simulink model "polysync_simulink"  (R2017a)
settings: Solver=FixedStepDiscrete  StartTime=0.0  StopTime=10.0  FixedStep=0.01  RelTol=1e-3
libraries: simulink x1, PolySyncLibrary x1
settings Model: Creator=laptopuser  LastModifiedBy=laptopuser
settings DataIOCC: SaveOutput=off  SignalLogging=off  DSMLogging=off  SaveTime=off
settings OptimizationCC: DefaultParameterBehavior=Inlined  UseDivisionForNetSlopeComputation=on  UseFloatMulNetSlope=on  InlineInvariantSignals=on  PassReuseOutputArgsThreshold=0  EfficientFloat2IntCast=on
settings DebuggingCC: ParameterTunabilityLossMsg=error
settings HardwareCC: ProdBitPerLong=64  ProdHWDeviceType=Intel->x86-64 (Linux 64)
settings SFSimCC: SimCustomHeaderCode="#include \"MwPsTypes.hpp\""  MATLABDynamicMemAlloc=off
settings RTWCC: GenerateReport=on  BuildConfiguration=Debug  LaunchReport=on  TargetLang=C++
settings CodeAppCC: ForceParamTrailComments=on  OperatorAnnotations=on  MATLABSourceComments=on
settings GRTTargetCC: TargetLangStandard=C++03 (ISO)

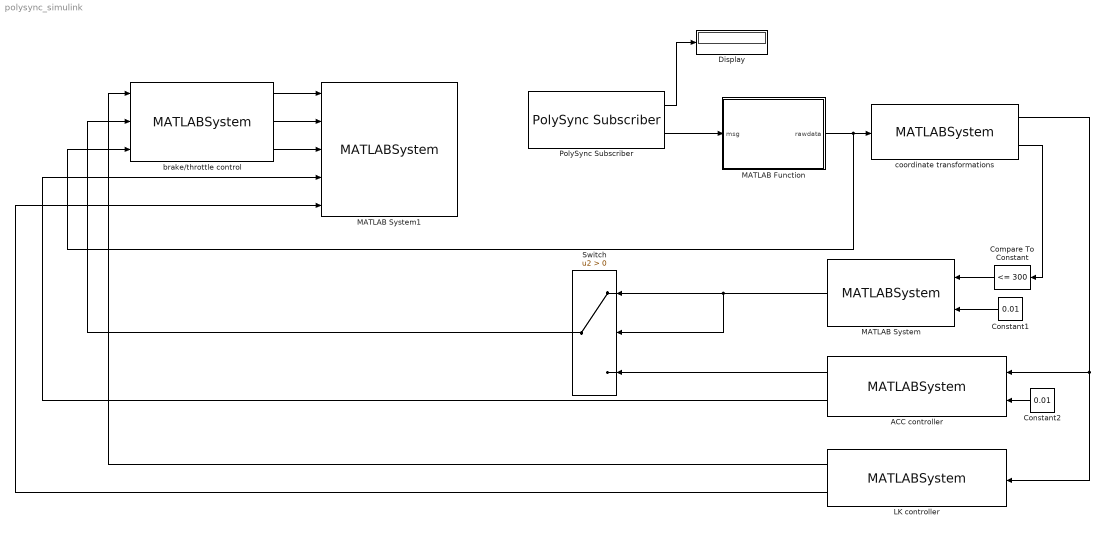
== system polysync_simulink ==
  ACC controller : MATLABSystem  System=acc_pcis_controller  M=1800  f0bar=74.63  f1bar=40.59  vl=26/3.6  v_des=28/3.6  H_x=diag([1 0.001])  f_x=[-28/3.6;0]  H_u=0.0001  f_u=0  K_i=50  sol_opts=struct( 'DataType', 'double', 'MaxIter', 200, 'FeasibilityTol', 1e-6, 'IntegrityChecks', true )  SimulateUsing=Code generation
      mask Type: acc_pcis_controller
      mask Display:
      | disp('acc_pcis_controller');
      | port_label('input',1,'lk_acc_state');
      | port_label('input',2,'dt');
      | port_label('output',1,'F_w');
      | port_label('output',2,'control_info');
  Compare To Constant : simulink/Logic and Bit Operations/Compare To Constant  relop=<=  const=300  OutDataTypeStr=boolean
  Constant1 : Constant  Value=0.01
  Constant2 : Constant  Value=0.01
  Display : Display
  LK controller : MATLABSystem  System=lk_pcis_controller  M=1800  lf=1.2  lr=1.650  Caf=140000  Car=120000  Iz=3270.0  H_x=diag([1 0 0.5 0])  f_x=[0;0;0;0]  H_u=0.25  f_u=0  sol_opts=struct( 'DataType', 'double', 'MaxIter', 200, 'FeasibilityTol', 1e-6, 'IntegrityChecks', true )  SimulateUsing=Code generation
      mask Type: lk_pcis_controller
      mask Display:
      | disp('lk_pcis_controller');
      | port_label('input',1,'lk_state');
      | port_label('output',1,'delta_f');
      | port_label('output',2,'control_info');
  MATLAB Function : MATLAB Function  TreatAsAtomicUnit=on
  MATLAB System : MATLABSystem  System=brake_ramp  end_ramp=2000  end_time=10  SimulateUsing=Code generation
      mask Type: brake_ramp
      mask Display:
      | disp('brake_ramp');
      | port_label('input',1,'is_active');
      | port_label('input',2,'dt');
      | port_label('output',1,'braking');
  MATLAB System1 : MATLABSystem  System=polysync_publisher  SimulateUsing=Code generation
      mask Type: polysync_publisher
      mask Display:
      | disp('polysync_publisher');
      | port_label('input',1,'steering');
      | port_label('input',2,'throttle');
      | port_label('input',3,'brake');
      | port_label('input',4,'cinfo_acc');
      | port_label('input',5,'cinfo_lk');
  PolySync Subscriber : PolySyncLibrary/PolySync Subscriber  MessageType=PlatformMotionMessage  SourceGuid=0  SensorId=0  SensorType=0
      settings: SourceProductName=PolySync
  Switch : Switch  Criteria=u2 > Threshold
  brake/throttle control : MATLABSystem  System=car_inputs  wheel_rad=0.392  trans_eff=0.79  steer_ratio=16.51  brake_gain=150/3000  inv_engine_map_file=inverse_engine_map.mat  SimulateUsing=Code generation
      mask Type: car_inputs
      mask Display:
      | disp('car_inputs');
      | port_label('input',1,'delta_f');
      | port_label('input',2,'F_w');
      | port_label('input',3,'rawdata');
      | port_label('output',1,'steering_angle');
      | port_label('output',2,'throttle');
      | port_label('output',3,'braking');
  coordinate transformations : MATLABSystem  System=road  lat0=42.30095833  long0=-83.69758056  h0=1  pathfile=/home/laptopuser/mkz/mcity/mcity_outer.ascii  circular=1  N_path=3  N_interp=10  dt=0.1  SimulateUsing=Code generation
      mask Type: road
      mask Display:
      | disp('road');
      | port_label('input',1,'data');
      | port_label('output',1,'lk_acc_state');
      | port_label('output',2,'road_left');
  wires:
  PolySync Subscriber/2 -> MATLAB Function/1(msg)
  MATLAB Function/1(rawdata) -> coordinate transformations/1, brake/throttle control/3
  coordinate transformations/1 -> LK controller/1, ACC controller/1
  Compare To Constant/1 -> MATLAB System/1
  coordinate transformations/2 -> Compare To Constant/1
  Constant1/1 -> MATLAB System/2
  Constant2/1 -> ACC controller/2
  MATLAB System/1 -> Switch/2, Switch/1
  Switch/1 -> brake/throttle control/2
  ACC controller/1 -> Switch/3
  LK controller/1 -> brake/throttle control/1
  brake/throttle control/1 -> MATLAB System1/1
  brake/throttle control/2 -> MATLAB System1/2
  brake/throttle control/3 -> MATLAB System1/3
  ACC controller/2 -> MATLAB System1/4
  LK controller/2 -> MATLAB System1/5
  PolySync Subscriber/1 -> Display/1

== matlab function polysync_simulink/MATLAB Function ==
  data: msg input; rawdata output Bus: DataBus
function rawdata = fcn(msg)
    rawdata.latitude = msg.Latitude;			% radians
    rawdata.longitude = msg.Longitude;          % radians
    rawdata.el = msg.Altitude;					% m
    rawdata.Yaw = msg.Heading;					% radians
    rawdata.YawRate = msg.RotationRate(3);		% rad/s
    rawdata.Vx = msg.Velocity(1);				% m/s
    rawdata.Vy = msg.Velocity(2);				% m/s
    rawdata.x_CG = -0.99;						% m
    rawdata.y_CG = NaN;							% m
    rawdata.steer_L1 = NaN;
    rawdata.steer_R1 = NaN;
    rawdata.Alpha_L1 = NaN;
    rawdata.Alpha_R1 = NaN;
    rawdata.Fy_L1 = NaN;
    rawdata.Fy_R1 = NaN;
    rawdata.Fz_L1 = NaN;
    rawdata.Fz_R1 = NaN;
    rawdata.Fx  = NaN;
    rawdata.Gear_CL = NaN;
    rawdata.RGear_Tr = NaN;
    rawdata.AV_Eng = 0;     					% rpm
    rawdata.Throttle = 0;						% [0, 1]
    rawdata.Throttle_Eng = NaN;			
    rawdata.M_EngOut = NaN;
    rawdata.AVy_L1 = 0;							% rpm
    rawdata.AVy_L2 = 0;
    rawdata.AVy_R1 = 0;
    rawdata.AVy_R2 = 0;
    rawdata.My_Dr_L1 = NaN;
    rawdata.My_Dr_L2 = NaN;
    rawdata.My_Dr_R1 = NaN;
    rawdata.My_Dr_R2 = NaN;
    rawdata.F_pedal = 0;
    rawdata.Bk_pedal = 0;
